simulink model "controller"  (R2023b)
settings: Solver=FixedStepAuto  StartTime=0.0  StopTime=100  FixedStep=1/100  RelTol=1e-3
undefined symbols (not defined in the file or in its folder): MAX_TORQUE, MAX_TORQUE_REVERSE
settings Model: Creator=DAUIN-Win10  LastModifiedBy=RSKALA
settings OptimizationCC: ReuseModelBlockBuffer=off
settings DebuggingCC: UnconnectedInputMsg=warning  UnconnectedOutputMsg=warning  UnconnectedLineMsg=warning
settings ModelReferenceCC: EnableRefExpFcnMdlSchedulingChecks=on
settings RTWCC: DLArmComputeVersion=19.05

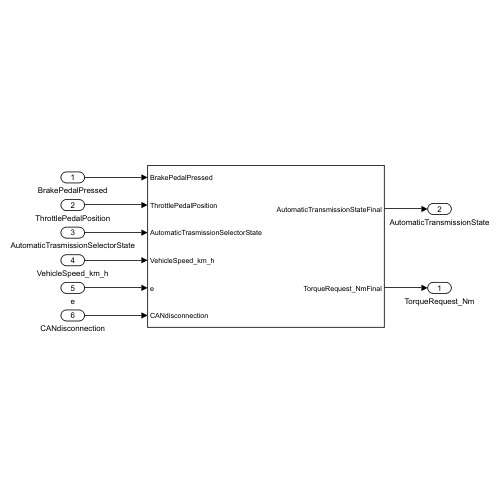
[thumbnail: Simulink's stored preview of the top-level diagram]
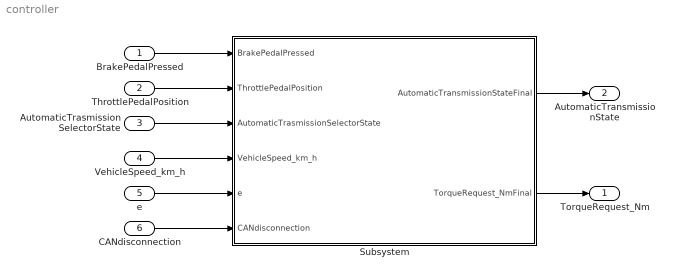
== system controller ==
  BrakePedalPressed : Inport  OutDataTypeStr=boolean
  ThrottlePedalPosition : Inport  Port=2  OutDataTypeStr=single
  AutomaticTrasmissionSelectorState : Inport  Port=3  OutDataTypeStr=Enum: TransmissionState
  VehicleSpeed_km_h : Inport  Port=4  OutDataTypeStr=single  Unit=km/h
  e : Inport  Port=5  OutDataTypeStr=single  Unit=km/h
  CANdisconnection : Inport  Port=6
  Subsystem : Subsystem
  TorqueRequest_Nm : Outport  OutDataTypeStr=single  Unit=N*m
  AutomaticTransmissionState : Outport  Port=2  OutDataTypeStr=Enum: TransmissionState
  wires:
  BrakePedalPressed/1 -> Subsystem/1(BrakePedalPressed)
  ThrottlePedalPosition/1 -> Subsystem/2(ThrottlePedalPosition)
  AutomaticTrasmissionSelectorState/1 -> Subsystem/3(AutomaticTrasmissionSelectorState)
  VehicleSpeed_km_h/1 -> Subsystem/4(VehicleSpeed_km_h)
  e/1 -> Subsystem/5(e)
  Subsystem/1(AutomaticTransmissionStateFinal) -> AutomaticTransmissionState/1
  Subsystem/2(TorqueRequest_NmFinal) -> TorqueRequest_Nm/1
  CANdisconnection/1 -> Subsystem/6(CANdisconnection)

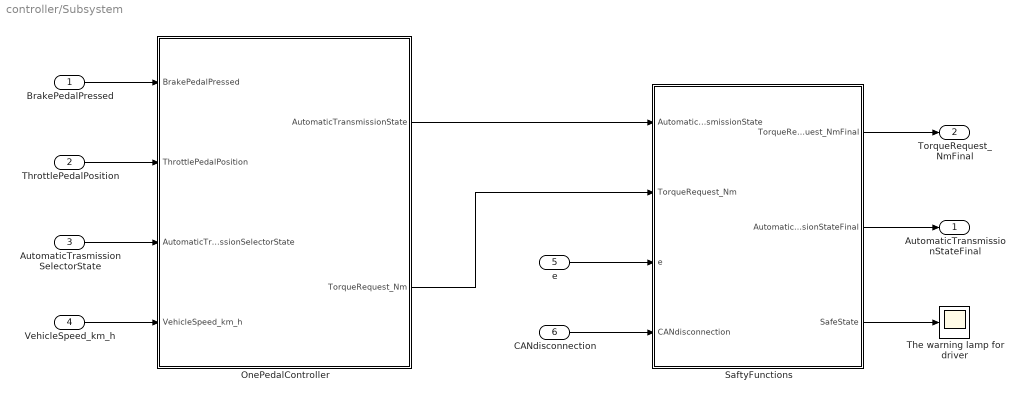
== system controller/Subsystem ==
  BrakePedalPressed : Inport  OutDataTypeStr=boolean
  ThrottlePedalPosition : Inport  Port=2  OutDataTypeStr=single
  AutomaticTrasmissionSelectorState : Inport  Port=3  OutDataTypeStr=Enum: TransmissionState
  VehicleSpeed_km_h : Inport  Port=4  OutDataTypeStr=single  Unit=km/h
  e : Inport  Port=5  OutDataTypeStr=single  Unit=km/h
  CANdisconnection : Inport  Port=6
  OnePedalController : Stateflow chart  TreatAsAtomicUnit=on
  SaftyFunctions : Stateflow chart  TreatAsAtomicUnit=on
      settings: PortSchema="{\"entries\":[{\"content\":{\"sides\":[{\"content\":{\"connectorIds\":[\"In1\",\"In2\",\"In4\",\"In3\"]},\"type\":\"ConnectorPlacement.EquallySpacedRectSide\",\"uuid\":\"7fe74ee5-44b1-4d05-a413-f8cbf6cc4146\"},{\"content\":{\"connectorIds\":[\"Out1\",\"Out2\",\"Out3\"],\"side\":\"RIGHT\"},\"type\":\"ConnectorPlacement.EquallySpacedRectSide\",\"uuid\":\"213ffcbc-04cb-45d6-b82c-0aa6f7f2fafd\"},{\"content\":{\"side\":\"TOP\"},\"type\":\"ConnectorPlacement.EquallySpacedRectSide\",\"uuid\":\"fb1fe60a-13ea-4390-8839-03c13817aaf9\"},{\"content\":{\"side\":\"BOTTOM\"},\"type\":\"ConnectorPlacement.EquallySpacedRectSide\",\"uuid\":\"05eed5e2-92b4-4d65-939e-09ec5391c094\"}]},\"type\":\"ConnectorPlacement.EquallySpacedConnector\",\"uuid\":\"3e98ccd8-4ab9-4b74-b636-0629ec9fe3f2\"}],\"packageUris\":[\"http://schema.mathworks.com/mf0/Connector/R2020b\"],\"version\":\"1.0\"}"
  The warning lamp for driver : Scope
  AutomaticTransmissionStateFinal : Outport  OutDataTypeStr=Enum: TransmissionState
  TorqueRequest_NmFinal : Outport  Port=2  OutDataTypeStr=single  Unit=N*m
  wires:
  ThrottlePedalPosition/1 -> OnePedalController/2(ThrottlePedalPosition)
  SaftyFunctions/1(TorqueRequest_NmFinal) -> TorqueRequest_NmFinal/1
  BrakePedalPressed/1 -> OnePedalController/1(BrakePedalPressed)
  AutomaticTrasmissionSelectorState/1 -> OnePedalController/3(AutomaticTrasmissionSelectorState)
  VehicleSpeed_km_h/1 -> OnePedalController/4(VehicleSpeed_km_h)
  CANdisconnection/1 -> SaftyFunctions/3(CANdisconnection)
  SaftyFunctions/2(AutomaticTransmissionStateFinal) -> AutomaticTransmissionStateFinal/1
  OnePedalController/1(AutomaticTransmissionState) -> SaftyFunctions/1(AutomaticTransmissionState)
  OnePedalController/2(TorqueRequest_Nm) -> SaftyFunctions/2(TorqueRequest_Nm)
  SaftyFunctions/3(SafeState) -> The warning lamp for driver/1
  e/1 -> SaftyFunctions/4(e)

== stateflow chart controller/Subsystem/SaftyFunctions ==
  state StateStateON
    du:
    AutomaticTransmissionStateFinal=TransmissionState.Neutral
    TorqueRequest_NmFinal=0
    SafeState=1
  state SafeStateOFF
    du:
    TorqueRequest_NmFinal=TorqueRequest_Nm
    AutomaticTransmissionStateFinal=AutomaticTransmissionState
    SafeState=0
  (default) -> StateStateON
  SafeStateOFF -> StateStateON : [abs(e)>=0.02||CANdisconnection==1]
  StateStateON -> SafeStateOFF : [abs(e)<=0.02&&CANdisconnection==0]
  data: AutomaticTransmissionState input; TorqueRequest_Nm input; CANdisconnection input; e input; TorqueRequest_NmFinal output; AutomaticTransmissionStateFinal output; SafeState output

== stateflow chart controller/Subsystem/OnePedalController ==
  state P
    en:
    AutomaticTransmissionState=TransmissionState.Park;
    du:
    TorqueRequest_Nm=0;
  state B
    en:
    AutomaticTransmissionState=TransmissionState.Brake;
    state Accelerate
      du:
      TorqueRequest_Nm=MAX_TORQUE*(3/2)*(ThrottlePedalPosition-(1/3));
    state Stop
      en:
      TorqueRequest_Nm=0;
    state Decelerate
      du:
      TorqueRequest_Nm=-MAX_TORQUE*(1-3*ThrottlePedalPosition);
    (default) -> Accelerate
    Stop -> Accelerate : [ThrottlePedalPosition>=1/3]
    Accelerate -> Decelerate : [ThrottlePedalPosition<=(1/3)]
    Decelerate -> Accelerate [order 2] : [ThrottlePedalPosition>(1/3)]
    Decelerate -> Stop [order 1] : [VehicleSpeed_km_h<=0]
  state N
    en:
    AutomaticTransmissionState=TransmissionState.Neutral;
    du:
    TorqueRequest_Nm=0;
  state R
    en:
    AutomaticTransmissionState=TransmissionState.Reverse;
    du:
    TorqueRequest_Nm=ThrottlePedalPosition*-MAX_TORQUE_REVERSE;
  state D
    en:
    AutomaticTransmissionState=TransmissionState.Drive;
    du:
    TorqueRequest_Nm=ThrottlePedalPosition*MAX_TORQUE;
  (default) -> P
  P -> N : [AutomaticTrasmissionSelectorState~=TransmissionState.Park&BrakePedalPressed==1]
  N -> P [order 1] : [AutomaticTrasmissionSelectorState==TransmissionState.Park&BrakePedalPressed==1&abs(VehicleSpeed_km_h)<5]
  N -> D [order 2] : [AutomaticTrasmissionSelectorState==TransmissionState.Drive||AutomaticTrasmissionSelectorState==TransmissionState.Brake&BrakePedalPressed==1&VehicleSpeed_km_h>-5]
  R -> N : [AutomaticTrasmissionSelectorState~=TransmissionState.Reverse]
  D -> N [order 2] : [AutomaticTrasmissionSelectorState==TransmissionState.Neutral || AutomaticTrasmissionSelectorState==TransmissionState.Reverse || AutomaticTrasmissionSelectorState==TransmissionState.Park]
  D -> B [order 1] : [ ThrottlePedalPosition>(1/3)&AutomaticTrasmissionSelectorState==TransmissionState.Brake]
  N -> R [order 3] : [AutomaticTrasmissionSelectorState==TransmissionState.Reverse&BrakePedalPressed==1&VehicleSpeed_km_h<5]
  B -> D : [AutomaticTrasmissionSelectorState~=TransmissionState.Brake]
  data: BrakePedalPressed input boolean; ThrottlePedalPosition input single; AutomaticTrasmissionSelectorState input Enum: TransmissionState; VehicleSpeed_km_h input single; AutomaticTransmissionState output Enum: TransmissionState; TorqueRequest_Nm output single; MAX_TORQUE_REVERSE parameter; MAX_TORQUE parameter
